simulink model "AgPVmodel_626"  (R2023b)
settings: Solver=VariableStepAuto  StartTime=0.0  StopTime=Tsim  RelTol=1e-3
undefined symbols (not defined in the file or in its folder): params, PVparams
libraries: fl_lib x31, nesl_utility x26, fl_ps_legacy_lib x4, ee_lib x4, spsPVArrayLib x2, batteryecm_lib x1, spsCurrentMeasurementLib x1, spsSeriesRLCBranchLib x1, spsVoltageMeasurementLib x1, sps_lib x1
settings Model: Creator=akoer  LastModifiedBy=akoer
settings DebuggingCC: SignalInfNanChecking=error

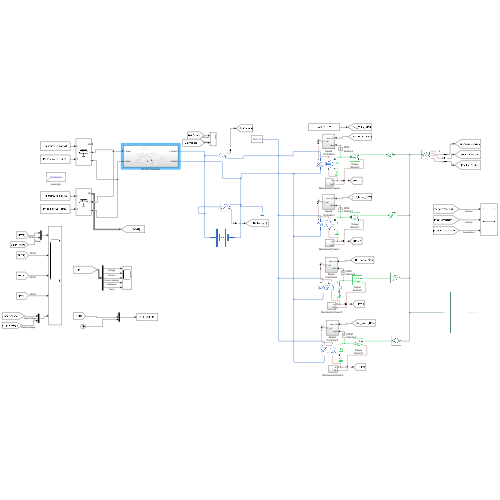
[thumbnail: Simulink's stored preview of the top-level diagram]
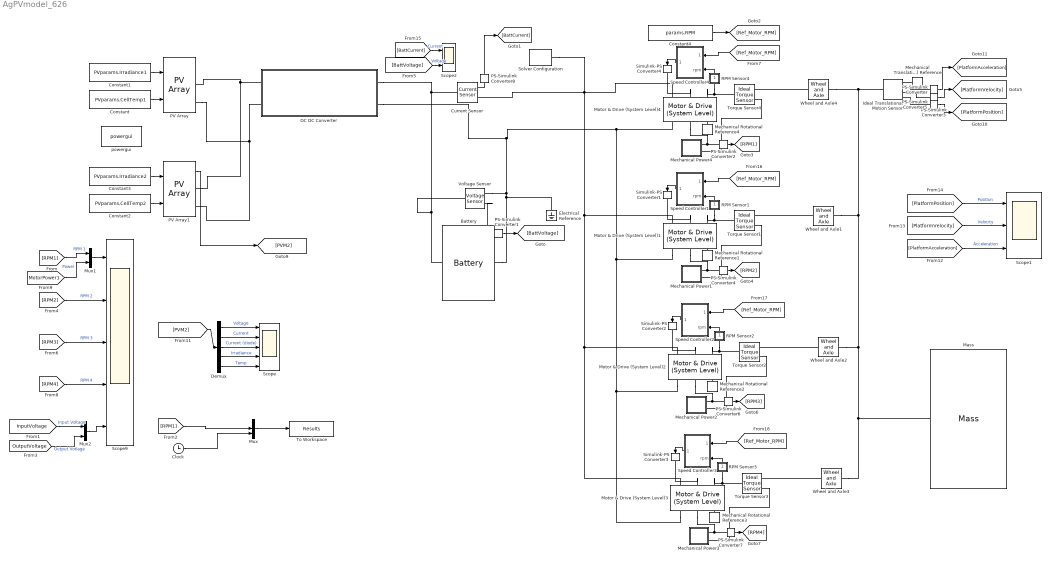
== system AgPVmodel_626 ==
  Battery : batteryecm_lib/Battery  Vnom=48 V  prm_dir=simscape.enum.battery.prm_dir.disabled  R1_dis=2 Ohm  R1_ch=2 Ohm  R1=2 Ohm  prm_AH=simscape.enum.battery.prm_AH.infinite  AH=50 A*hr  V1=11.5 V  AH1=25 A*hr  prm_R2=simscape.enum.battery.prm_R2.disabled  R2=2000 Ohm  Tmeas=298.15 K  charge_measurement_port=simscape.enum.battery.enable.no  prm_dyn=simscape.enum.battery.prm_dyn.off  Rp1=0.005 Ohm  tau1=30 s  Rp2=0.005 Ohm  tau2=30 s  Rp3=0.005 Ohm  tau3=30 s  Rp4=0.005 Ohm  tau4=30 s  Rp5=0.005 Ohm  tau5=30 s  prm_fade=simscape.enum.battery.prm_fade.disabled  N_fade=100  AH_fade=45 A*hr  R1_fade=2.02 Ohm  R1_ch_fade=2.02 Ohm  V1_fade=10.35 V  prm_age=simscape.enum.battery.prm_age.disabled  prm_age_OCV=simscape.enum.battery.prm_age_OCV.OCV  OCV_age=0.9  SOC_age=60  Tmeas_age=298.15 K  delta_time_age_vec=[0] d  temperature_age_vec=[273] K  OCV_scaling_age=2.2134e6  OCV_offset_age=1.632e6  temp_exp_age=0.515833569 V  t_exp_age=0.75  Vnom_T2=12 V  R1_T2=2.2 Ohm  R1_T2_dis=2.2 Ohm  R1_T2_ch=2.2 Ohm  V1_T2=11.4 V  R2_T2=2200 Ohm  Rp1_T2=0.005 Ohm  tau1_T2=30 s  Rp2_T2=0.005 Ohm  tau2_T2=30 s  Rp3_T2=0.005 Ohm  tau3_T2=30 s  Rp4_T2=0.005 Ohm  tau4_T2=30 s  Rp5_T2=0.005 Ohm  tau5_T2=30 s  Tmeas2=273.15 K  thermal_port=simscape.enum.thermaleffects.omit  thermal_mass=30000 J/K  i_specify=off  i_priority=None  i=0 A  i_nominal_specify=off  i_nominal_unit=A  i_nominal_value=1  v_specify=on  v_priority=None  v=48 V  v_nominal_specify=off  v_nominal_unit=V  v_nominal_value=1  charge_specify=off  charge_priority=High  charge=50 A*hr  charge_nominal_specify=off  charge_nominal_unit=A*hr  charge_nominal_value=1  num_cycles_specify=off  num_cycles_priority=High  num_cycles=0  num_cycles_nominal_specify=off  num_cycles_nominal_unit=1  num_cycles_nominal_value=1  temperature_specify=off  temperature_priority=High  temperature=298.15 K  temperature_nominal_specify=off  temperature_nominal_unit=K  temperature_nominal_value=1
      settings: LibrarySourceBlock=batt_lib/Cells/Battery
  Clock : Clock
  Constant : Constant  Value=PVparams.CellTemp1
  Constant1 : Constant  Value=PVparams.Irradiance1
  Constant2 : Constant  Value=PVparams.CellTemp2
  Constant3 : Constant  Value=PVparams.Irradiance2
  Constant4 : Constant  Value=params.RPM
  Current Sensor : fl_lib/Electrical/Electrical Sensors/Current Sensor
  DC DC Converter : Subsystem
  Demux : Demux  Outputs=5
  Electrical Reference : fl_lib/Electrical/Electrical Elements/Electrical Reference
  Ideal Translational Motion Sensor : fl_lib/Mechanical/Mechanical Sensors/Ideal Translational Motion Sensor  reference=foundation.enum.MeasurementReference.difference  acceleration_port=true  velocity_port=true  position_port=true  offset=0 m
      settings: InternalSimscapePortConfiguration="{\"Bottom\":[],\"Left\":[{\"id\":\"R\",\"label\":\"R\",\"type\":\"foundation.mechanical.translational.translational\"}],\"Right\":[{\"id\":\"C\",\"label\":\"C\",\"type\":\"foundation.mechanical.translational.translational\"},{\"id\":\"A\",\"label\":\"A\",\"type\":\"output\"},{\"id\":\"V\",\"label\":\"V\",\"type\":\"output\"},{\"id\":\"P\",\"label\":\"P\",\"type\":\"output\"}],\"Top\":[]}"
  Mass : fl_lib/Mechanical/Translational Elements/Mass  mass=13 kg  num_ports=foundation.enum.numPorts2.one  v_specify=off  v_priority=High  v=0 m/s  v_nominal_specify=off  v_nominal_unit=m/s  v_nominal_value=1  f_specify=off  f_priority=None  f=0 N  f_nominal_specify=off  f_nominal_unit=N  f_nominal_value=1
  Mechanical Rotational Reference{1..4} (4 alike) : fl_lib/Mechanical/Rotational Elements/Mechanical Rotational Reference
  Mechanical Translational Reference : fl_lib/Mechanical/Translational Elements/Mechanical Translational Reference
  Mechanical Power1 : Subsystem
  Mechanical Power2 : Subsystem
  Mechanical Power3 : Subsystem
  Mechanical Power4 : Subsystem
  Motor & Drive (System Level)1 : ee_lib/Electromechanical/Motor & Drive (System Level)  torque_speed_param=ee.enum.electromech.envelope.tabulated2D  overtorque_param=ee.enum.electromech.overtorque.no  T_t=[.09, .08, .07, 0] N*m  T_t_intermittent=[.36, .32, .28, 0] N*m  T_t_2D=[.09, .09, .09; .08, .08, .08; .07, .07, .07; 0, 0, 0] N*m  T_t_intermittent_2D=[.36, .36, .36; .32, .32, .32; .28, .28, .28; 0, 0, 0] N*m  w_t=[0, 3750, 7500, 8000] rpm  vdc_t=[6, 12, 24] V  torque_max=0.1 N*m  power_max=30 W  torque_max_intermittent=0.4 N*m  power_max_intermittent=120 W  time_overtorque=30 s  time_recover=60 s  Tc=0.02 s  EnableSwitch=false  losses_param=1  eff=100  w_eff=3750 rpm  T_eff=0.08 N*m  Piron=0 W  Pbase=0 W  w_eff_vec=[-8000, -4000, 0, 4000, 8000] rpm  T_eff_vec=[0, .03, .06, .09] N*m  v_eff_vec=[100, 250, 400] V  losses_mat=[1.49, 1.67, 2.21, 3.1; .42, .69, 1.14, 2.03; .06, .24, .78, 1.68; .42, .69, 1.14, 2.03; 1.49, 1.67, 2.21, 3.1] W  efficiency_mat=[95, 95, 95, 95; 95, 95, 95, 95; 95, 95, 95, 95; 95, 95, 95, 95; 95, 95, 95, 95]  losses_mat_3D=ones(5, 4, 3) W  efficiency_mat_3D=95 * ones(5, 4, 3)  Res=0 Ohm  enable_fault=simscape.enum.onoff.off  fault_condition=1  fault_threshold=0.5  J=5e-6 kg*m^2  lam=1e-5 N*m*s/rad  speed0=0 rpm  faulted_specify=off  faulted_priority=None  faulted=0  faulted_nominal_specify=off  faulted_nominal_unit=1  faulted_nominal_value=1  isSwitchedOff_specify=off  isSwitchedOff_priority=None  isSwitchedOff=0  isSwitchedOff_nominal_specify=off  isSwitchedOff_nominal_unit=1  isSwitchedOff_nominal_value=1  torqueLimitContinuous_specify=off  torqueLimitContinuous_priority=None  torqueLimitContinuous=0 N*m  torqueLimitContinuous_nominal_specify=off  torqueLimitContinuous_nominal_unit=N*m  torqueLimitContinuous_nominal_value=1  alpha=3.93e-3 1/K  Tmeas=25 degC  Tmeas2=125 degC  losses_mat_T2=[1.49, 1.74, 2.49, 3.74; .42, .67, 1.42, 2.67; .06, .31, 1.06, 2.31; .42, .67, 1.42, 2.67; 1.49, 1.74, 2.49, 3.74] W  efficiency_mat_T2=[95, 95, 95, 95; 95, 95, 95, 95; 95, 95, 95, 95; 95, 95, 95, 95; 95, 95, 95, 95]  losses_mat_3D_T2=ones(5, 4, 3) W  efficiency_mat_3D_T2=95 * ones(5, 4, 3)  thermal_mass=100 J/K  initial_temperature=25 degC
  Motor & Drive (System Level)2 : ee_lib/Electromechanical/Motor & Drive (System Level)  torque_speed_param=ee.enum.electromech.envelope.tabulated2D  overtorque_param=ee.enum.electromech.overtorque.no  T_t=[.09, .08, .07, 0] N*m  T_t_intermittent=[.36, .32, .28, 0] N*m  T_t_2D=[.09, .09, .09; .08, .08, .08; .07, .07, .07; 0, 0, 0] N*m  T_t_intermittent_2D=[.36, .36, .36; .32, .32, .32; .28, .28, .28; 0, 0, 0] N*m  w_t=[0, 3750, 7500, 8000] rpm  vdc_t=[6, 12, 24] V  torque_max=0.1 N*m  power_max=30 W  torque_max_intermittent=0.4 N*m  power_max_intermittent=120 W  time_overtorque=30 s  time_recover=60 s  Tc=0.02 s  EnableSwitch=false  losses_param=1  eff=100  w_eff=3750 rpm  T_eff=0.08 N*m  Piron=0 W  Pbase=0 W  w_eff_vec=[-8000, -4000, 0, 4000, 8000] rpm  T_eff_vec=[0, .03, .06, .09] N*m  v_eff_vec=[100, 250, 400] V  losses_mat=[1.49, 1.67, 2.21, 3.1; .42, .69, 1.14, 2.03; .06, .24, .78, 1.68; .42, .69, 1.14, 2.03; 1.49, 1.67, 2.21, 3.1] W  efficiency_mat=[95, 95, 95, 95; 95, 95, 95, 95; 95, 95, 95, 95; 95, 95, 95, 95; 95, 95, 95, 95]  losses_mat_3D=ones(5, 4, 3) W  efficiency_mat_3D=95 * ones(5, 4, 3)  Res=0 Ohm  enable_fault=simscape.enum.onoff.off  fault_condition=1  fault_threshold=0.5  J=5e-6 kg*m^2  lam=1e-5 N*m*s/rad  speed0=0 rpm  faulted_specify=off  faulted_priority=None  faulted=0  faulted_nominal_specify=off  faulted_nominal_unit=1  faulted_nominal_value=1  isSwitchedOff_specify=off  isSwitchedOff_priority=None  isSwitchedOff=0  isSwitchedOff_nominal_specify=off  isSwitchedOff_nominal_unit=1  isSwitchedOff_nominal_value=1  torqueLimitContinuous_specify=off  torqueLimitContinuous_priority=None  torqueLimitContinuous=0 N*m  torqueLimitContinuous_nominal_specify=off  torqueLimitContinuous_nominal_unit=N*m  torqueLimitContinuous_nominal_value=1  alpha=3.93e-3 1/K  Tmeas=25 degC  Tmeas2=125 degC  losses_mat_T2=[1.49, 1.74, 2.49, 3.74; .42, .67, 1.42, 2.67; .06, .31, 1.06, 2.31; .42, .67, 1.42, 2.67; 1.49, 1.74, 2.49, 3.74] W  efficiency_mat_T2=[95, 95, 95, 95; 95, 95, 95, 95; 95, 95, 95, 95; 95, 95, 95, 95; 95, 95, 95, 95]  losses_mat_3D_T2=ones(5, 4, 3) W  efficiency_mat_3D_T2=95 * ones(5, 4, 3)  thermal_mass=100 J/K  initial_temperature=25 degC
  Motor & Drive (System Level)3 : ee_lib/Electromechanical/Motor & Drive (System Level)  torque_speed_param=ee.enum.electromech.envelope.tabulated2D  overtorque_param=ee.enum.electromech.overtorque.no  T_t=[.09, .08, .07, 0] N*m  T_t_intermittent=[.36, .32, .28, 0] N*m  T_t_2D=[.09, .09, .09; .08, .08, .08; .07, .07, .07; 0, 0, 0] N*m  T_t_intermittent_2D=[.36, .36, .36; .32, .32, .32; .28, .28, .28; 0, 0, 0] N*m  w_t=[0, 3750, 7500, 8000] rpm  vdc_t=[6, 12, 24] V  torque_max=0.1 N*m  power_max=30 W  torque_max_intermittent=0.4 N*m  power_max_intermittent=120 W  time_overtorque=30 s  time_recover=60 s  Tc=0.02 s  EnableSwitch=false  losses_param=1  eff=100  w_eff=3750 rpm  T_eff=0.08 N*m  Piron=0 W  Pbase=0 W  w_eff_vec=[-8000, -4000, 0, 4000, 8000] rpm  T_eff_vec=[0, .03, .06, .09] N*m  v_eff_vec=[100, 250, 400] V  losses_mat=[1.49, 1.67, 2.21, 3.1; .42, .69, 1.14, 2.03; .06, .24, .78, 1.68; .42, .69, 1.14, 2.03; 1.49, 1.67, 2.21, 3.1] W  efficiency_mat=[95, 95, 95, 95; 95, 95, 95, 95; 95, 95, 95, 95; 95, 95, 95, 95; 95, 95, 95, 95]  losses_mat_3D=ones(5, 4, 3) W  efficiency_mat_3D=95 * ones(5, 4, 3)  Res=0 Ohm  enable_fault=simscape.enum.onoff.off  fault_condition=1  fault_threshold=0.5  J=5e-6 kg*m^2  lam=1e-5 N*m*s/rad  speed0=0 rpm  faulted_specify=off  faulted_priority=None  faulted=0  faulted_nominal_specify=off  faulted_nominal_unit=1  faulted_nominal_value=1  isSwitchedOff_specify=off  isSwitchedOff_priority=None  isSwitchedOff=0  isSwitchedOff_nominal_specify=off  isSwitchedOff_nominal_unit=1  isSwitchedOff_nominal_value=1  torqueLimitContinuous_specify=off  torqueLimitContinuous_priority=None  torqueLimitContinuous=0 N*m  torqueLimitContinuous_nominal_specify=off  torqueLimitContinuous_nominal_unit=N*m  torqueLimitContinuous_nominal_value=1  alpha=3.93e-3 1/K  Tmeas=25 degC  Tmeas2=125 degC  losses_mat_T2=[1.49, 1.74, 2.49, 3.74; .42, .67, 1.42, 2.67; .06, .31, 1.06, 2.31; .42, .67, 1.42, 2.67; 1.49, 1.74, 2.49, 3.74] W  efficiency_mat_T2=[95, 95, 95, 95; 95, 95, 95, 95; 95, 95, 95, 95; 95, 95, 95, 95; 95, 95, 95, 95]  losses_mat_3D_T2=ones(5, 4, 3) W  efficiency_mat_3D_T2=95 * ones(5, 4, 3)  thermal_mass=100 J/K  initial_temperature=25 degC
  Motor & Drive (System Level)4 : ee_lib/Electromechanical/Motor & Drive (System Level)  torque_speed_param=ee.enum.electromech.envelope.tabulated2D  overtorque_param=ee.enum.electromech.overtorque.no  T_t=[.09, .08, .07, 0] N*m  T_t_intermittent=[.36, .32, .28, 0] N*m  T_t_2D=[.09, .09, .09,.09; .08, .08, .08,.08; .07, .07, .07,.07; 0, 0, 0,0] N*m  T_t_intermittent_2D=[.36, .36, .36; .32, .32, .32; .28, .28, .28; 0, 0, 0] N*m  w_t=[0, 3750, 7500, 8000] rpm  vdc_t=[6, 12, 24, 48] V  torque_max=0.1 N*m  power_max=30 W  torque_max_intermittent=0.4 N*m  power_max_intermittent=120 W  time_overtorque=30 s  time_recover=60 s  Tc=0.02 s  EnableSwitch=false  losses_param=1  eff=100  w_eff=3750 rpm  T_eff=0.08 N*m  Piron=0 W  Pbase=0 W  w_eff_vec=[-8000, -4000, 0, 4000, 8000] rpm  T_eff_vec=[0, .03, .06, .09] N*m  v_eff_vec=[100, 250, 400] V  losses_mat=[1.49, 1.67, 2.21, 3.1; .42, .69, 1.14, 2.03; .06, .24, .78, 1.68; .42, .69, 1.14, 2.03; 1.49, 1.67, 2.21, 3.1] W  efficiency_mat=[95, 95, 95, 95; 95, 95, 95, 95; 95, 95, 95, 95; 95, 95, 95, 95; 95, 95, 95, 95]  losses_mat_3D=ones(5, 4, 3) W  efficiency_mat_3D=95 * ones(5, 4, 3)  Res=0 Ohm  enable_fault=simscape.enum.onoff.off  fault_condition=1  fault_threshold=0.5  J=5e-6 kg*m^2  lam=1e-5 N*m*s/rad  speed0=0 rpm  faulted_specify=off  faulted_priority=None  faulted=0  faulted_nominal_specify=off  faulted_nominal_unit=1  faulted_nominal_value=1  isSwitchedOff_specify=off  isSwitchedOff_priority=None  isSwitchedOff=0  isSwitchedOff_nominal_specify=off  isSwitchedOff_nominal_unit=1  isSwitchedOff_nominal_value=1  torqueLimitContinuous_specify=off  torqueLimitContinuous_priority=None  torqueLimitContinuous=0 N*m  torqueLimitContinuous_nominal_specify=off  torqueLimitContinuous_nominal_unit=N*m  torqueLimitContinuous_nominal_value=1  alpha=3.93e-3 1/K  Tmeas=25 degC  Tmeas2=125 degC  losses_mat_T2=[1.49, 1.74, 2.49, 3.74; .42, .67, 1.42, 2.67; .06, .31, 1.06, 2.31; .42, .67, 1.42, 2.67; 1.49, 1.74, 2.49, 3.74] W  efficiency_mat_T2=[95, 95, 95, 95; 95, 95, 95, 95; 95, 95, 95, 95; 95, 95, 95, 95; 95, 95, 95, 95]  losses_mat_3D_T2=ones(5, 4, 3) W  efficiency_mat_3D_T2=95 * ones(5, 4, 3)  thermal_mass=100 J/K  initial_temperature=25 degC
  Mux : Mux  Inputs=3
  Mux1 : Mux  Inputs=2
  Mux2 : Mux  Inputs=2
  PS-Simulink Converter{,1..8} (9 alike) : nesl_utility/PS-Simulink Converter  PhysicalDomain=network_engine_domain  SubClassName=ps_output  LeftPortType=input  RightPortType=output  PseudoPeriodic=off  Frequencies=[]  VectorFormat=inherit  Unit=inherit  AffineConversion=off
  PV Array : spsPVArrayLib/PV Array  Npar=PVparams.Parallel1  Nser=PVparams.Series1  PlotType=array @ 1000 W/m2 & specified temperatures  S_vec="[ 1000  500  100 ]"  Temp_C_vec="[ 45 25  ]"  ModuleName=American Solar Wholesale ASW-185M  PlotWhenSelected=off  Pm=185.13  Ncell=72  Voc=44.6  Isc=5.37  Vm=37.4  Im=4.95  beta_Voc_pc=-0.38595  alpha_Isc_pc=0.043594  beta_Voc=-0.17213  alpha_Isc=0.002341  IL=5.3768  I0=4.1873e-10  nI=1.0375  Rsh=226.7768  Rs=0.28792  RobustModel=off  RobustCellTemperature=313.3991  BAL=on  Tc=1e-6  Tfilter=5e-5
  PV Array1 : spsPVArrayLib/PV Array  Npar=PVparams.Parallel2  Nser=PVparams.Series2  PlotType=array @ 1000 W/m2 & specified temperatures  S_vec="[ 1000  500  100 ]"  Temp_C_vec="[ 45 25  ]"  ModuleName=American Solar Wholesale ASW-185M  PlotWhenSelected=off  Pm=185.13  Ncell=72  Voc=44.6  Isc=5.37  Vm=37.4  Im=4.95  beta_Voc_pc=-0.38595  alpha_Isc_pc=0.043594  beta_Voc=-0.17213  alpha_Isc=0.002341  IL=5.3768  I0=4.1873e-10  nI=1.0375  Rsh=226.7768  Rs=0.28792  RobustModel=off  RobustCellTemperature=313.3991  BAL=on  Tc=1e-6  Tfilter=5e-5
  RPM Sensor1 : Subsystem
      mask Display: disp('S')
  RPM Sensor2 : Subsystem
      mask Display: disp('S')
  RPM Sensor3 : Subsystem
      mask Display: disp('S')
  RPM Sensor4 : Subsystem
      mask Display: disp('S')
  Scope : Scope  NumInputPorts=5
  Scope1 : Scope  NumInputPorts=3
  Scope2 : Scope  NumInputPorts=2
  Scope9 : Scope  NumInputPorts=5
  Simulink-PS Converter{1..4} (4 alike) : nesl_utility/Simulink-PS Converter  PhysicalDomain=network_engine_domain  SubClassName=ps_input  LeftPortType=input  RightPortType=output  PseudoPeriodic=off  Frequencies=[]  NoiseDistribution=none  NoiseParameters=[]  Unit=1  AffineConversion=off  FilteringAndDerivatives=provide  SimscapeFilterOrder=1  InputFilterTimeConstant=0.001  UdotUserProvided=0
  Solver Configuration : nesl_utility/Solver Configuration  PhysicalDomain=network_engine_domain  SubClassName=solver  LeftPortType=input  RightPortType=generic  Tones=[]  Harmonics=[]  SimulateNoise=off  Profile=off  UseLocalSampling=off  EnableSwitchedLinearOptims=on  FrequencyDomain=off  UseCCode=off  RelTol=0.001  AbsTol=0.001  MinStep=1e-09  ToWorkspace=off  RevertToSquareIcSolve=off  NumHomotopyIterations=100  PhasorMode=off  PhasorModeNumHarmonics=1  ConsistencySolver=NEWTON_XTOL_AFTER_FTOL  IndexReductionMethod=DerivativeReplacement  DoDC=off  ResidualTolerance=1e-09  ConsistencyTolSource=GLOBAL  ConsistencyAbsTol=0.001  ConsistencyRelTol=0.001  ConsistencyTolFactor=0.001  UseLocalSolver=off  LocalSolverChoice=NE_BACKWARD_EULER_ADVANCER  ResolveIndetEquations=on  FunctionEvalNumThread=1  LocalSolverSampleTime=0.001  DoFixedCost=off  MaxNonlinIter=3  MaxModeIter=2  ComputeImpulses=off  ImpulseIterations=2  LinearAlgebra=auto  LinearAlgebraNumThread=0  EquationFormulation=NE_TIME_EF  DelaysMemoryBudget=2048  AutomaticFiltering=on  FilteringTimeConstant=0.001  PartitionStorageMethod=AS_NEEDED  PartitionMemoryBudget=1024  PartitionMethod=ROBUST  MultibodyUseLocalSolver=off  MultibodyLocalSolverChoice=ODE1  MultibodyLocalSolverSampleTime=0.001
  Speed Controller1 : Subsystem
  Speed Controller2 : Subsystem
  Speed Controller3 : Subsystem
  Speed Controller4 : Subsystem
  To Workspace : ToWorkspace  VariableName=Results  SampleTime=-1
  Torque Sensor{1..4} (4 alike) : fl_lib/Mechanical/Mechanical Sensors/Ideal Torque Sensor
  Voltage Sensor : fl_lib/Electrical/Electrical Sensors/Voltage Sensor
  Wheel and Axle{1..4} (4 alike) : fl_lib/Mechanical/Mechanisms/Wheel and Axle  R=.125 m  or=1  t_specify=off  t_priority=None  t=0 N*m  t_nominal_specify=off  t_nominal_unit=N*m  t_nominal_value=1  f_specify=off  f_priority=None  f=0 N  f_nominal_specify=off  f_nominal_unit=N  f_nominal_value=1
  powergui : sps_lib/powergui  Priority=1  SimulationMode=Continuous  SampleTime=50e-4  frequency=60  Iterations=50  frequencyindice=0  Pbase=100e6  ErrMax=1e-4  UnitsV=kV  UnitsW=MW  buscounter=0  FunctionMessages=off  echomessages=off  EnableUseOfTLC=off  CurrentSourceSwitches=off  DisableSnubberDevices=off  DisableRonSwitches=off  DisableVfSwitches=off  DisplayEquations=off  AutomaticDiscreteSolvers=off  SolverType=Tustin/Backward Euler (TBE)  Interpol=off  ExternalGateDelay=off  methode=off  Ts=100  x0status=blocks  SPID=on  SwTol=0  HookPort=off  NonlinearTolerance=1e-4  nMaxIteration=100  ContinueOnMaxIteration=off  RestoreLinks=warning  ResistiveCurrentMeasurement=off  Frange=[0:2:500]  Ylog=off  Xlog=on  ShowGrid=off  save=off  variable=ZData  structure=0  ZoomFFT=off  StartTime=0.0  cycles=1  DisplayStyle=1  fundamental=60  FreqAxis=off  MaxFrequency=1000  frequencyindicesteady=1  RmsSteady=1  display=off
  wires:
  Constant/1 -> PV Array/2
  Constant1/1 -> PV Array/1
  Constant3/1 -> PV Array1/1
  Constant2/1 -> PV Array1/2
  Mux/1 -> To Workspace/1
  [RPM1] -> Mux/2
  [RPM1] -> Mux1/1  "RPM 1"
  Clock/1 -> Mux/3
  Mux1/1 -> Scope9/1
  [RPM2] -> Scope9/2  "RPM 2"
  [RPM4] -> Scope9/4  "RPM 4"
  PV Array1/1 -> [PVM2]
  [RPM3] -> Scope9/3  "RPM 3"
  [PVM2] -> Demux/1
  Demux/1 -> Scope/1  "Voltage"
  Demux/2 -> Scope/2  "Current"
  Demux/3 -> Scope/3  "Current (diode)"
  Demux/4 -> Scope/4  "Irradiance"
  Demux/5 -> Scope/5  "Temp"
  [InputVoltage] -> Mux2/1  "Input Voltage"
  Mux2/1 -> Scope9/5
  Constant4/1 -> [Ref_Motor_RPM]
  [MotorPower1] -> Mux1/2  "Power"
  PS-Simulink Converter/1 -> [PlatformAcceleration]
  PS-Simulink Converter3/1 -> [PlatformVelocity]
  PS-Simulink Converter5/1 -> [PlatformPosition]
  [PlatformPosition] -> Scope1/1  "Position"
  [PlatformVelocity] -> Scope1/2  "Velocity"
  [PlatformAcceleration] -> Scope1/3  "Acceleration"
  PS-Simulink Converter1/1 -> [BattVoltage]
  PS-Simulink Converter8/1 -> [BattCurrent]
  [BattCurrent] -> Scope2/1  "Current"
  RPM Sensor1/1(rpm) -> Speed Controller1/2(rpm)
  PS-Simulink Converter4/1 -> [RPM2]
  Speed Controller1/1(T_ref) -> Simulink-PS Converter1/1
  [Ref_Motor_RPM] -> Speed Controller1/1(rpm_ref)
  Speed Controller2/1(T_ref) -> Simulink-PS Converter2/1
  [Ref_Motor_RPM] -> Speed Controller2/1(rpm_ref)
  RPM Sensor2/1(rpm) -> Speed Controller2/2(rpm)
  PS-Simulink Converter6/1 -> [RPM3]
  Speed Controller3/1(T_ref) -> Simulink-PS Converter3/1
  [Ref_Motor_RPM] -> Speed Controller3/1(rpm_ref)
  RPM Sensor3/1(rpm) -> Speed Controller3/2(rpm)
  PS-Simulink Converter7/1 -> [RPM4]
  Speed Controller4/1(T_ref) -> Simulink-PS Converter4/1
  [Ref_Motor_RPM] -> Speed Controller4/1(rpm_ref)
  RPM Sensor4/1(rpm) -> Speed Controller4/2(rpm)
  PS-Simulink Converter2/1 -> [RPM1]
  [OutputVoltage] -> Mux2/2  "Output Votlage"
  [BattVoltage] -> Scope2/2  "Voltage"
  connections:
  PV Array1/RConn2 -- DC DC Converter/LConn2 -- PV Array/RConn2
  Ideal Translational Motion Sensor/LConn1 -- Mass/LConn1 -- Wheel and Axle3/RConn1 -- Wheel and Axle2/RConn1 -- Wheel and Axle1/RConn1 -- Wheel and Axle4/RConn1
  Mechanical Translational Reference/LConn1 -- Ideal Translational Motion Sensor/RConn1
  Ideal Translational Motion Sensor/RConn2 -- PS-Simulink Converter/LConn1
  Ideal Translational Motion Sensor/RConn3 -- PS-Simulink Converter3/LConn1
  Electrical Reference/LConn1 -- Battery/RConn1 -- Motor & Drive (System Level)2/RConn1 -- Motor & Drive (System Level)3/RConn1 -- Motor & Drive (System Level)1/RConn1 -- Motor & Drive (System Level)4/RConn1 -- DC DC Converter/RConn2 -- Voltage Sensor/RConn2
  Battery/LConn1 -- Voltage Sensor/LConn1 -- DC DC Converter/RConn1 -- Current Sensor/LConn1
  PS-Simulink Converter5/LConn1 -- Ideal Translational Motion Sensor/RConn4
  Voltage Sensor/RConn1 -- PS-Simulink Converter1/LConn1
  Current Sensor/RConn1 -- PS-Simulink Converter8/LConn1
  Solver Configuration/RConn1 -- Current Sensor/RConn2 -- Motor & Drive (System Level)2/LConn1 -- Motor & Drive (System Level)3/LConn1 -- Motor & Drive (System Level)1/LConn1 -- Motor & Drive (System Level)4/LConn1
  Mechanical Power1/RConn1 -- Motor & Drive (System Level)1/RConn2 -- PS-Simulink Converter4/LConn1
  Motor & Drive (System Level)1/LConn3 -- Torque Sensor1/LConn1 -- RPM Sensor1/LConn1
  Wheel and Axle1/LConn1 -- Torque Sensor1/RConn1
  Mechanical Rotational Reference1/LConn1 -- Motor & Drive (System Level)1/RConn3
  Torque Sensor1/RConn2 -- Mechanical Power1/RConn2
  Motor & Drive (System Level)1/LConn2 -- Simulink-PS Converter1/RConn1
  Mechanical Power2/RConn1 -- Motor & Drive (System Level)2/RConn2 -- PS-Simulink Converter6/LConn1
  Motor & Drive (System Level)2/LConn3 -- Torque Sensor2/LConn1 -- RPM Sensor2/LConn1
  Torque Sensor2/RConn2 -- Mechanical Power2/RConn2
  Mechanical Rotational Reference2/LConn1 -- Motor & Drive (System Level)2/RConn3
  Wheel and Axle2/LConn1 -- Torque Sensor2/RConn1
  Motor & Drive (System Level)2/LConn2 -- Simulink-PS Converter2/RConn1
  Mechanical Power3/RConn1 -- Motor & Drive (System Level)3/RConn2 -- PS-Simulink Converter7/LConn1
  Motor & Drive (System Level)3/LConn3 -- Torque Sensor3/LConn1 -- RPM Sensor3/LConn1
  Torque Sensor3/RConn2 -- Mechanical Power3/RConn2
  Mechanical Rotational Reference3/LConn1 -- Motor & Drive (System Level)3/RConn3
  Wheel and Axle3/LConn1 -- Torque Sensor3/RConn1
  Motor & Drive (System Level)3/LConn2 -- Simulink-PS Converter3/RConn1
  Mechanical Power4/RConn1 -- Motor & Drive (System Level)4/RConn2 -- PS-Simulink Converter2/LConn1
  Motor & Drive (System Level)4/LConn3 -- Torque Sensor4/LConn1 -- RPM Sensor4/LConn1
  Torque Sensor4/RConn2 -- Mechanical Power4/RConn2
  Mechanical Rotational Reference4/LConn1 -- Motor & Drive (System Level)4/RConn3
  Wheel and Axle4/LConn1 -- Torque Sensor4/RConn1
  Motor & Drive (System Level)4/LConn2 -- Simulink-PS Converter4/RConn1
  PV Array1/RConn1 -- DC DC Converter/LConn1 -- PV Array/RConn1

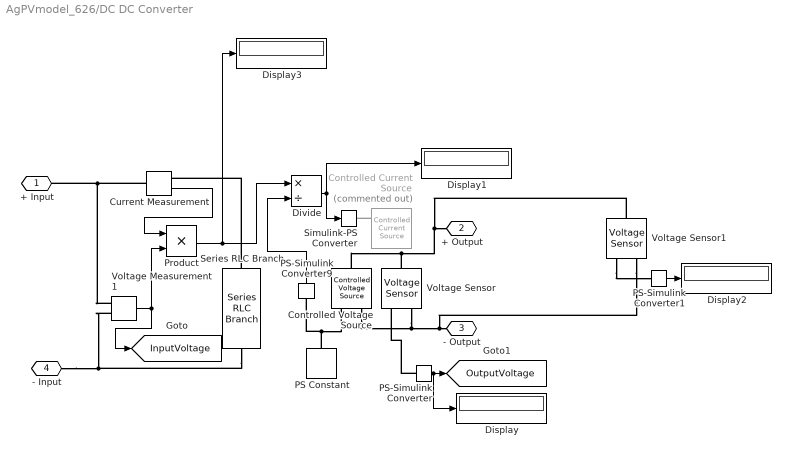
== system AgPVmodel_626/DC DC Converter ==
  Controlled Current Source : fl_lib/Electrical/Electrical Sources/Controlled Current Source  Commented=on
  Controlled Voltage Source : fl_lib/Electrical/Electrical Sources/Controlled Voltage Source
  Current Measurement : spsCurrentMeasurementLib/Current Measurement  PhasorSimulation=off  OutputType=Complex  PSBequivalent=0
  Display{,1..3} (4 alike) : Display
  Divide : Product  Inputs=*/
  PS Constant : fl_lib/Physical Signals/Sources/PS Constant  constant=ConverterParams.OutputVoltage V
  PS-Simulink Converter : nesl_utility/PS-Simulink Converter  PhysicalDomain=network_engine_domain  SubClassName=ps_output  LeftPortType=input  RightPortType=output  PseudoPeriodic=off  Frequencies=[]  VectorFormat=inherit  Unit=inherit  AffineConversion=off
  PS-Simulink Converter1 : nesl_utility/PS-Simulink Converter  PhysicalDomain=network_engine_domain  SubClassName=ps_output  LeftPortType=input  RightPortType=output  PseudoPeriodic=off  Frequencies=[]  VectorFormat=inherit  Unit=inherit  AffineConversion=off
  PS-Simulink Converter9 : nesl_utility/PS-Simulink Converter  PhysicalDomain=network_engine_domain  SubClassName=ps_output  LeftPortType=input  RightPortType=output  PseudoPeriodic=off  Frequencies=[]  VectorFormat=inherit  Unit=inherit  AffineConversion=off
  Product : Product
  Series RLC Branch : spsSeriesRLCBranchLib/Series RLC Branch  LConnTagsString=__new0  RConnTagsString=__new0  BranchType=R  Resistance=1  Inductance=1e-3  SetiL0=off  InitialCurrent=0  Capacitance=1e-6  Setx0=off  InitialVoltage=0  Measurements=None
  Simulink-PS Converter : nesl_utility/Simulink-PS Converter  PhysicalDomain=network_engine_domain  SubClassName=ps_input  LeftPortType=input  RightPortType=output  PseudoPeriodic=off  Frequencies=[]  NoiseDistribution=none  NoiseParameters=[]  Unit=1  AffineConversion=off  FilteringAndDerivatives=provide  SimscapeFilterOrder=1  InputFilterTimeConstant=0.001  UdotUserProvided=0
  Voltage Measurement1 : spsVoltageMeasurementLib/Voltage Measurement  PhasorSimulation=off  OutputType=Complex  PSBequivalent=0
  Voltage Sensor : fl_lib/Electrical/Electrical Sensors/Voltage Sensor
  Voltage Sensor1 : fl_lib/Electrical/Electrical Sensors/Voltage Sensor
  + Input : PMIOPort  Side=Left
  + Output : PMIOPort  Port=2  Side=Right
  - Output : PMIOPort  Port=3  Side=Right
  - Input : PMIOPort  Port=4  Side=Left
  tag scope: InputVoltage=global, OutputVoltage=global
  wires:
  Divide/1 -> Simulink-PS Converter/1, Display1/1
  Voltage Measurement1/1 -> Product/2, [InputVoltage]
  PS-Simulink Converter9/1 -> Divide/2
  Product/1 -> Display3/1, Divide/1
  Current Measurement/1 -> Product/1
  PS-Simulink Converter/1 -> Display/1, [OutputVoltage]
  PS-Simulink Converter1/1 -> Display2/1
  connections:
  PS Constant/RConn1 -- Controlled Voltage Source/RConn1 -- PS-Simulink Converter9/LConn1
  Voltage Measurement1/LConn1 -- Current Measurement/LConn1 -- + Input/RConn1
  Controlled Current Source/RConn1 -- Simulink-PS Converter/RConn1
  Series RLC Branch/LConn1 -- Current Measurement/RConn1
  Voltage Sensor1/LConn1 -- Voltage Sensor/LConn1 -- Controlled Voltage Source/LConn1 -- + Output/RConn1
  Controlled Voltage Source/RConn2 -- Voltage Sensor1/RConn2 -- - Output/RConn1 -- Voltage Sensor/RConn2
  - Input/RConn1 -- Voltage Measurement1/LConn2 -- Series RLC Branch/RConn1
  PS-Simulink Converter/LConn1 -- Voltage Sensor/RConn1
  Voltage Sensor1/RConn1 -- PS-Simulink Converter1/LConn1

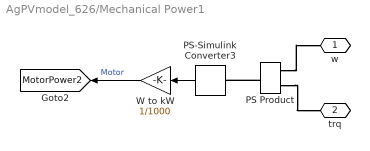
== system AgPVmodel_626/Mechanical Power1 ==
  " W to kW " : Gain  Gain=1/1000
  PS Product : fl_ps_legacy_lib/Legacy Physical Signals/Functions/PS Product
  PS-Simulink Converter3 : nesl_utility/PS-Simulink Converter  PhysicalDomain=network_engine_domain  SubClassName=ps_output  LeftPortType=input  RightPortType=output  PseudoPeriodic=off  Frequencies=[]  VectorFormat=1-D array  Unit=W  AffineConversion=off
  w : PMIOPort  Side=Right
  trq : PMIOPort  Port=2  Side=Right
  tag scope: MotorPower2=global
  wires:
  " W to kW "/1 -> [MotorPower2]  "Motor"
  PS-Simulink Converter3/1 -> " W to kW "/1
  connections:
  PS Product/LConn1 -- trq/RConn1
  PS Product/LConn2 -- w/RConn1
  PS Product/RConn1 -- PS-Simulink Converter3/LConn1

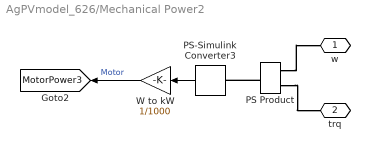
== system AgPVmodel_626/Mechanical Power2 ==
  " W to kW " : Gain  Gain=1/1000
  PS Product : fl_ps_legacy_lib/Legacy Physical Signals/Functions/PS Product
  PS-Simulink Converter3 : nesl_utility/PS-Simulink Converter  PhysicalDomain=network_engine_domain  SubClassName=ps_output  LeftPortType=input  RightPortType=output  PseudoPeriodic=off  Frequencies=[]  VectorFormat=1-D array  Unit=W  AffineConversion=off
  w : PMIOPort  Side=Right
  trq : PMIOPort  Port=2  Side=Right
  tag scope: MotorPower3=global
  wires:
  " W to kW "/1 -> [MotorPower3]  "Motor"
  PS-Simulink Converter3/1 -> " W to kW "/1
  connections:
  PS Product/LConn1 -- trq/RConn1
  PS Product/LConn2 -- w/RConn1
  PS Product/RConn1 -- PS-Simulink Converter3/LConn1

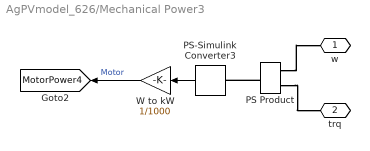
== system AgPVmodel_626/Mechanical Power3 ==
  " W to kW " : Gain  Gain=1/1000
  PS Product : fl_ps_legacy_lib/Legacy Physical Signals/Functions/PS Product
  PS-Simulink Converter3 : nesl_utility/PS-Simulink Converter  PhysicalDomain=network_engine_domain  SubClassName=ps_output  LeftPortType=input  RightPortType=output  PseudoPeriodic=off  Frequencies=[]  VectorFormat=1-D array  Unit=W  AffineConversion=off
  w : PMIOPort  Side=Right
  trq : PMIOPort  Port=2  Side=Right
  tag scope: MotorPower4=global
  wires:
  " W to kW "/1 -> [MotorPower4]  "Motor"
  PS-Simulink Converter3/1 -> " W to kW "/1
  connections:
  PS Product/LConn1 -- trq/RConn1
  PS Product/LConn2 -- w/RConn1
  PS Product/RConn1 -- PS-Simulink Converter3/LConn1

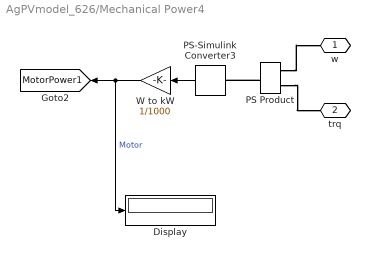
== system AgPVmodel_626/Mechanical Power4 ==
  " W to kW " : Gain  Gain=1/1000
  Display : Display
  PS Product : fl_ps_legacy_lib/Legacy Physical Signals/Functions/PS Product
  PS-Simulink Converter3 : nesl_utility/PS-Simulink Converter  PhysicalDomain=network_engine_domain  SubClassName=ps_output  LeftPortType=input  RightPortType=output  PseudoPeriodic=off  Frequencies=[]  VectorFormat=1-D array  Unit=W  AffineConversion=off
  w : PMIOPort  Side=Right
  trq : PMIOPort  Port=2  Side=Right
  tag scope: MotorPower1=global
  wires:
  " W to kW "/1 -> Display/1, [MotorPower1]  "Motor"
  PS-Simulink Converter3/1 -> " W to kW "/1
  connections:
  PS Product/LConn1 -- trq/RConn1
  PS Product/LConn2 -- w/RConn1
  PS Product/RConn1 -- PS-Simulink Converter3/LConn1

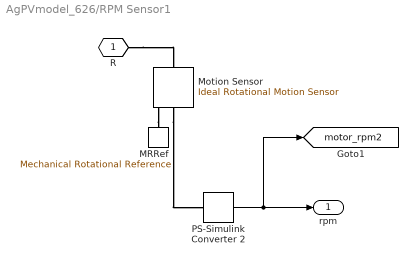
== system AgPVmodel_626/RPM Sensor1 ==
  MRRef : fl_lib/Mechanical/Rotational Elements/Mechanical Rotational Reference
  Motion Sensor : fl_lib/Mechanical/Mechanical Sensors/Ideal Rotational Motion Sensor  reference=foundation.enum.MeasurementReference.difference  acceleration_port=false  velocity_port=true  position_port=true  wrap_angle=simscape.enum.onoff.off  offset=0 rad
  PS-Simulink Converter 2 : nesl_utility/PS-Simulink Converter  PhysicalDomain=network_engine_domain  SubClassName=ps_output  LeftPortType=input  RightPortType=output  PseudoPeriodic=off  Frequencies=[]  VectorFormat=1-D array  Unit=rpm  AffineConversion=off
  R : PMIOPort  Side=Left
  rpm : Outport  VectorParamsAs1DForOutWhenUnconnected=off
  tag scope: motor_rpm2=global
  wires:
  PS-Simulink Converter 2/1 -> [motor_rpm2], rpm/1
  connections:
  R/RConn1 -- Motion Sensor/LConn1
  Motion Sensor/RConn1 -- MRRef/LConn1
  Motion Sensor/RConn2 -- PS-Simulink Converter 2/LConn1

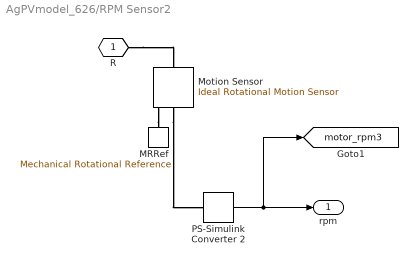
== system AgPVmodel_626/RPM Sensor2 ==
  MRRef : fl_lib/Mechanical/Rotational Elements/Mechanical Rotational Reference
  Motion Sensor : fl_lib/Mechanical/Mechanical Sensors/Ideal Rotational Motion Sensor  reference=foundation.enum.MeasurementReference.difference  acceleration_port=false  velocity_port=true  position_port=true  wrap_angle=simscape.enum.onoff.off  offset=0 rad
  PS-Simulink Converter 2 : nesl_utility/PS-Simulink Converter  PhysicalDomain=network_engine_domain  SubClassName=ps_output  LeftPortType=input  RightPortType=output  PseudoPeriodic=off  Frequencies=[]  VectorFormat=1-D array  Unit=rpm  AffineConversion=off
  R : PMIOPort  Side=Left
  rpm : Outport  VectorParamsAs1DForOutWhenUnconnected=off
  tag scope: motor_rpm3=global
  wires:
  PS-Simulink Converter 2/1 -> [motor_rpm3], rpm/1
  connections:
  R/RConn1 -- Motion Sensor/LConn1
  Motion Sensor/RConn1 -- MRRef/LConn1
  Motion Sensor/RConn2 -- PS-Simulink Converter 2/LConn1

== system AgPVmodel_626/RPM Sensor3 ==
  MRRef : fl_lib/Mechanical/Rotational Elements/Mechanical Rotational Reference
  Motion Sensor : fl_lib/Mechanical/Mechanical Sensors/Ideal Rotational Motion Sensor  reference=foundation.enum.MeasurementReference.difference  acceleration_port=false  velocity_port=true  position_port=true  wrap_angle=simscape.enum.onoff.off  offset=0 rad
  PS-Simulink Converter 2 : nesl_utility/PS-Simulink Converter  PhysicalDomain=network_engine_domain  SubClassName=ps_output  LeftPortType=input  RightPortType=output  PseudoPeriodic=off  Frequencies=[]  VectorFormat=1-D array  Unit=rpm  AffineConversion=off
  R : PMIOPort  Side=Left
  rpm : Outport  VectorParamsAs1DForOutWhenUnconnected=off
  tag scope: motor_rpm4=global
  wires:
  PS-Simulink Converter 2/1 -> [motor_rpm4], rpm/1
  connections:
  R/RConn1 -- Motion Sensor/LConn1
  Motion Sensor/RConn1 -- MRRef/LConn1
  Motion Sensor/RConn2 -- PS-Simulink Converter 2/LConn1

== system AgPVmodel_626/RPM Sensor4 ==
  MRRef : fl_lib/Mechanical/Rotational Elements/Mechanical Rotational Reference
  Motion Sensor : fl_lib/Mechanical/Mechanical Sensors/Ideal Rotational Motion Sensor  reference=foundation.enum.MeasurementReference.difference  acceleration_port=false  velocity_port=true  position_port=true  wrap_angle=simscape.enum.onoff.off  offset=0 rad
  PS-Simulink Converter 2 : nesl_utility/PS-Simulink Converter  PhysicalDomain=network_engine_domain  SubClassName=ps_output  LeftPortType=input  RightPortType=output  PseudoPeriodic=off  Frequencies=[]  VectorFormat=1-D array  Unit=rpm  AffineConversion=off
  R : PMIOPort  Side=Left
  rpm : Outport  VectorParamsAs1DForOutWhenUnconnected=off
  tag scope: motor_rpm1=global
  wires:
  PS-Simulink Converter 2/1 -> [motor_rpm1], rpm/1
  connections:
  R/RConn1 -- Motion Sensor/LConn1
  Motion Sensor/RConn1 -- MRRef/LConn1
  Motion Sensor/RConn2 -- PS-Simulink Converter 2/LConn1

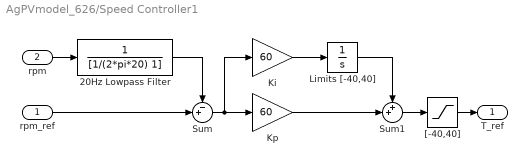
== system AgPVmodel_626/Speed Controller1 ==
  rpm_ref : Inport
  rpm : Inport  Port=2
  20Hz Lowpass Filter : TransferFcn  Denominator=[1/(2*pi*20) 1]
  Ki : Gain  Gain=60
  Kp : Gain  Gain=60
  Limits [-40,40] : Integrator  LimitOutput=on  UpperSaturationLimit=40  LowerSaturationLimit=-40
  Sum : Sum  Inputs=-+|
  Sum1 : Sum  Inputs=++|
  "[-40,40]" : Saturate  UpperLimit=400  LowerLimit=-400
  T_ref : Outport  VectorParamsAs1DForOutWhenUnconnected=off
  wires:
  "[-40,40]"/1 -> T_ref/1
  20Hz Lowpass Filter/1 -> Sum/1
  Limits [-40,40]/1 -> Sum1/1
  Kp/1 -> Sum1/2
  Ki/1 -> Limits [-40,40]/1
  Sum/1 -> Kp/1, Ki/1
  Sum1/1 -> "[-40,40]"/1
  rpm/1 -> 20Hz Lowpass Filter/1
  rpm_ref/1 -> Sum/2

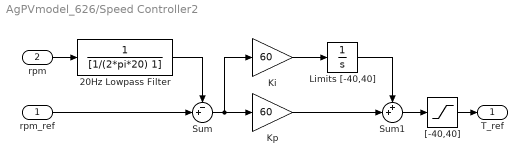
== system AgPVmodel_626/Speed Controller2 ==
  rpm_ref : Inport
  rpm : Inport  Port=2
  20Hz Lowpass Filter : TransferFcn  Denominator=[1/(2*pi*20) 1]
  Ki : Gain  Gain=60
  Kp : Gain  Gain=60
  Limits [-40,40] : Integrator  LimitOutput=on  UpperSaturationLimit=40  LowerSaturationLimit=-40
  Sum : Sum  Inputs=-+|
  Sum1 : Sum  Inputs=++|
  "[-40,40]" : Saturate  UpperLimit=400  LowerLimit=-400
  T_ref : Outport  VectorParamsAs1DForOutWhenUnconnected=off
  wires:
  "[-40,40]"/1 -> T_ref/1
  20Hz Lowpass Filter/1 -> Sum/1
  Limits [-40,40]/1 -> Sum1/1
  Kp/1 -> Sum1/2
  Ki/1 -> Limits [-40,40]/1
  Sum/1 -> Kp/1, Ki/1
  Sum1/1 -> "[-40,40]"/1
  rpm/1 -> 20Hz Lowpass Filter/1
  rpm_ref/1 -> Sum/2

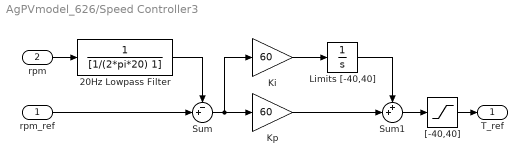
== system AgPVmodel_626/Speed Controller3 ==
  rpm_ref : Inport
  rpm : Inport  Port=2
  20Hz Lowpass Filter : TransferFcn  Denominator=[1/(2*pi*20) 1]
  Ki : Gain  Gain=60
  Kp : Gain  Gain=60
  Limits [-40,40] : Integrator  LimitOutput=on  UpperSaturationLimit=40  LowerSaturationLimit=-40
  Sum : Sum  Inputs=-+|
  Sum1 : Sum  Inputs=++|
  "[-40,40]" : Saturate  UpperLimit=400  LowerLimit=-400
  T_ref : Outport  VectorParamsAs1DForOutWhenUnconnected=off
  wires:
  "[-40,40]"/1 -> T_ref/1
  20Hz Lowpass Filter/1 -> Sum/1
  Limits [-40,40]/1 -> Sum1/1
  Kp/1 -> Sum1/2
  Ki/1 -> Limits [-40,40]/1
  Sum/1 -> Kp/1, Ki/1
  Sum1/1 -> "[-40,40]"/1
  rpm/1 -> 20Hz Lowpass Filter/1
  rpm_ref/1 -> Sum/2

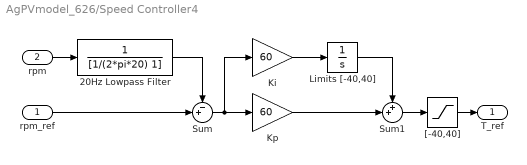
== system AgPVmodel_626/Speed Controller4 ==
  rpm_ref : Inport
  rpm : Inport  Port=2
  20Hz Lowpass Filter : TransferFcn  Denominator=[1/(2*pi*20) 1]
  Ki : Gain  Gain=60
  Kp : Gain  Gain=60
  Limits [-40,40] : Integrator  LimitOutput=on  UpperSaturationLimit=40  LowerSaturationLimit=-40
  Sum : Sum  Inputs=-+|
  Sum1 : Sum  Inputs=++|
  "[-40,40]" : Saturate  UpperLimit=400  LowerLimit=-400
  T_ref : Outport  VectorParamsAs1DForOutWhenUnconnected=off
  wires:
  "[-40,40]"/1 -> T_ref/1
  20Hz Lowpass Filter/1 -> Sum/1
  Limits [-40,40]/1 -> Sum1/1
  Kp/1 -> Sum1/2
  Ki/1 -> Limits [-40,40]/1
  Sum/1 -> Kp/1, Ki/1
  Sum1/1 -> "[-40,40]"/1
  rpm/1 -> 20Hz Lowpass Filter/1
  rpm_ref/1 -> Sum/2
